simulink model "system_sim"  (R2015b)
settings: Solver=ode45  StartTime=0.0  StopTime=100  RelTol=1e-3
InitFcn:
  | param
undefined symbols (not defined in the file or in its folder): ctrl, P
settings Model: Creator=beard  LastModifiedBy=magiccjae
settings DataIOCC: SaveFormat=Array  SignalLoggingSaveFormat=ModelDataLogs
settings OptimizationCC: ExpressionDepthLimit=2147483647  InitFltsAndDblsToZero=on
settings DebuggingCC: UnderspecifiedInitializationDetection=Classic  MergeDetectMultiDrivingBlocksExec=none  SolverPrmCheckMsg=warning  FcnCallInpInsideContextMsg=UseLocalSettings  StateNameClashWarn=warning
settings HardwareCC: ProdBitPerPointer=32  ProdLargestAtomicFloat=None  ProdIntDivRoundTo=Undefined  ProdEndianess=Unspecified  ProdWordSize=32  ProdHWDeviceType=32-bit Generic
settings GRTTargetCC: GeneratePreprocessorConditionals=Disable all  CombineOutputUpdateFcns=off  GRTInterface=on
settings ConfigComp: CovModelRefEnable=Off

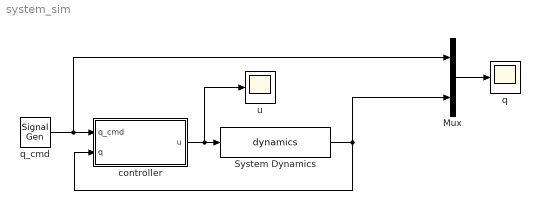
== system system_sim ==
  Mux : Mux  Inputs=2
  System Dynamics : S-Function  FunctionName=dynamics  Parameters=P  SFunctionDeploymentMode=off  EnableBusSupport=off
  controller : Subsystem
  q : Scope
  q_cmd : SignalGenerator  WaveForm=square  Frequency=.1
  u : Scope
  wires:
  controller/1(u) -> u/1, System Dynamics/1
  q_cmd/1 -> Mux/1, controller/1(q_cmd)
  Mux/1 -> q/1
  System Dynamics/1 -> Mux/2, controller/2(q)

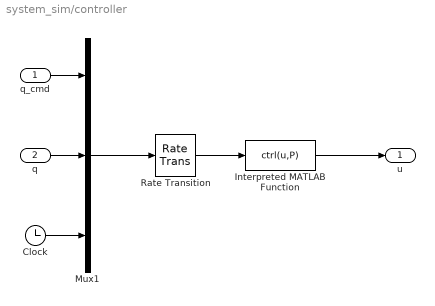
== system system_sim/controller ==
  q_cmd : Inport
  q : Inport  Port=2
  Clock : Clock
  Interpreted MATLAB Function : MATLABFcn  MATLABFcn=ctrl(u,P)  OutputDimensions=1
  Mux1 : Mux  Inputs=3
  Rate Transition : RateTransition  OutPortSampleTime=P.Ts
  u : Outport
  wires:
  Mux1/1 -> Rate Transition/1
  q_cmd/1 -> Mux1/1
  Interpreted MATLAB Function/1 -> u/1
  Clock/1 -> Mux1/3
  Rate Transition/1 -> Interpreted MATLAB Function/1
  q/1 -> Mux1/2
